simulink model "TwoLVSCSwitch_IGBT"  (R2018a)
settings: Solver=VariableStepAuto  StartTime=0.0  StopTime=0.5  RelTol=1e-3
values from neighbouring files (symbols this model uses):
  C = 1 / (C_pu * omega_base * Z_DC_base)    (= 0.000114731723891)    [ErlingInitialization.m]
  I_base = 2 * S_base / (3 * V_base)    (= 33.3333333333)    [ErlingInitialization.m]
  I_DC_base = S_base / V_DC_base    (= 25)    [ErlingInitialization.m]
  i_load = I_DC_base    (= 25)    [ErlingInitialization.m]
  K_CRCI = K_CRCP / tau    [ErlingInitialization.m]
  K_CRCP = 1 / (C_pu * omega_base * sqrt(tau * tau_eq))    [ErlingInitialization.m]
  K_i = R_pu / tau_eq    (= 16.6666666667)    [ErlingInitialization.m]
  K_p = L_pu / (omega_base * tau_eq)    (= 0.795774715459)    [ErlingInitialization.m]
  L = L_pu * Z_base / omega_base    (= 0.00572957795131)    [ErlingInitialization.m]
  L_pu = 0.15    [ErlingInitialization.m]
  R = R_pu * Z_base    (= 0.12)    [ErlingInitialization.m]
  tau_PWM = 1 / 10000    (= 0.0001)    [ErlingInitialization.m]
  Ts = 1e-6    (= 1e-06)    [ErlingInitialization.m]
  V_base = 400    [ErlingInitialization.m]
  V_DC_base = V_base * 2    (= 800)    [ErlingInitialization.m]
  V_DC_start = V_DC_base    (= 800)    [ErlingInitialization.m]
libraries: powerlib x17
settings Model: Creator=nartgnilre  LastModifiedBy=nartgnilre

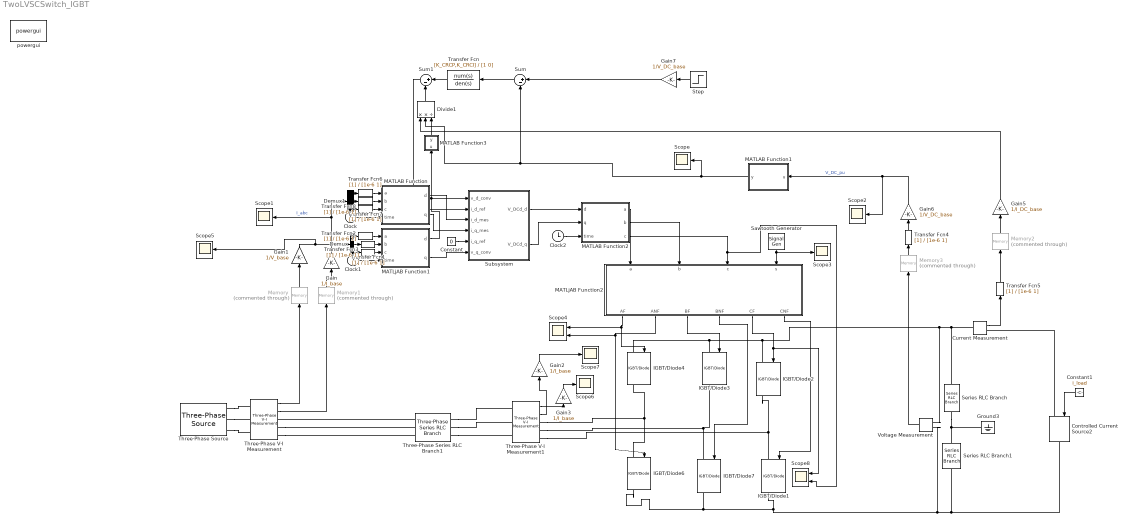
== system TwoLVSCSwitch_IGBT ==
  Clock : Clock
  Clock1 : Clock
  Clock2 : Clock
  Constant : Constant  Value=0
  Constant1 : Constant  Value=i_load
  Controlled Current Source2 : powerlib/Electrical Sources/Controlled Current Source  Initialize=on  Source_Type=AC  Amplitude=0  Phase=0  Frequency=0  Measurements=None
  Current Measurement : powerlib/Measurements/Current Measurement  PhasorSimulation=off  OutputType=Magnitude  PSBequivalent=0
  Demux : Demux  Outputs=3
  Demux1 : Demux  Outputs=3
  Divide1 : Product  Inputs=**/
  Gain : Gain  Gain=1/I_base
  Gain1 : Gain  Gain=1/V_base
  Gain2 : Gain  Gain=1/I_base
  Gain3 : Gain  Gain=1/I_base
  Gain5 : Gain  Gain=1/I_DC_base
  Gain6 : Gain  Gain=1/V_DC_base
  Gain7 : Gain  Gain=1/V_DC_base
  Ground3 : powerlib/Elements/Ground  LConnTagsString=a
  IGBT/Diode{1..4,6..7} (6 alike) : powerlib/Power Electronics/IGBT//Diode  Ron=1e-5  Rs=1e5  Cs=inf  Measurements=on
  MATLAB Function : MATLAB Function  TreatAsAtomicUnit=on
  MATLAB Function1 : MATLAB Function  TreatAsAtomicUnit=on
  MATLAB Function2 : MATLAB Function  TreatAsAtomicUnit=on
  MATLAB Function3 : MATLAB Function  TreatAsAtomicUnit=on
  MATLjAB Function1 : MATLAB Function  TreatAsAtomicUnit=on
  MATLjAB Function2 : MATLAB Function  TreatAsAtomicUnit=on
  Memory : Memory  Commented=through  InitialCondition=V_base
  Memory1 : Memory  Commented=through  InitialCondition=I_base
  Memory2 : Memory  Commented=through  InitialCondition=I_base
  Memory3 : Memory  Commented=through  InitialCondition=V_base
  Sawtooth Generator : SignalGenerator  WaveForm=sawtooth  Frequency=1/tau_PWM
  Scope{,1..3,5..7} (7 alike) : Scope
  Scope4 : Scope  NumInputPorts=2
  Scope8 : Scope  NumInputPorts=2
  Series RLC Branch : powerlib/Elements/Series RLC Branch  LConnTagsString=__new0  RConnTagsString=__new0  BranchType=C  Resistance=1  Inductance=1e-3  SetiL0=off  InitialCurrent=0  Capacitance=2*C  Setx0=on  InitialVoltage=V_DC_start/2  Measurements=None
  Series RLC Branch1 : powerlib/Elements/Series RLC Branch  LConnTagsString=__new0  RConnTagsString=__new0  BranchType=C  Resistance=1  Inductance=1e-3  SetiL0=off  InitialCurrent=0  Capacitance=2*C  Setx0=on  InitialVoltage=-V_DC_start/2  Measurements=None
  Step : Step  Time=0.4  Before=V_DC_start*1.2  After=V_DC_start*1.3  SampleTime=0
  Subsystem : Subsystem
  Sum : Sum  Inputs=|+-
  Sum1 : Sum  Inputs=|+-
  Three-Phase Series RLC Branch1 : powerlib/Elements/Three-Phase Series RLC Branch  LConnTagsString=A|B|C  RConnTagsString=A|B|C  BranchType=RL  Resistance=R  Inductance=L  Capacitance=0  Measurements=Branch voltages and currents
  Three-Phase V-I Measurement : powerlib/Measurements/Three-Phase V-I Measurement  VoltageMeasurement=phase-to-ground  SetLabelV=off  LabelV=Vabc  Vpu=off  VpuLL=off  CurrentMeasurement=yes  SetLabelI=off  LabelI=Iabc  Ipu=off  Pbase=S_base  Vbase=V_base  OutputType=Complex  PhasorSimulation=off  PSBequivalent=0
  Three-Phase V-I Measurement1 : powerlib/Measurements/Three-Phase V-I Measurement  VoltageMeasurement=phase-to-ground  SetLabelV=off  LabelV=Vabc  Vpu=off  VpuLL=off  CurrentMeasurement=yes  SetLabelI=off  LabelI=Iabc  Ipu=off  Pbase=S_base  Vbase=V_base  OutputType=Complex  PhasorSimulation=off  PSBequivalent=0
  Three-Phase Source : powerlib/Electrical Sources/Three-Phase Source  InternalConnection=Yg  VoltagePhases=off  Voltage=V_base*sqrt(3)/sqrt(2)  PhaseAngle=90  Voltage_phases=[25e3 25e3 25e3]/sqrt(3)  PhaseAngles_phases=[0 -120 +120]  Frequency=50  NonIdealSource=off  SpecifyImpedance=off  Resistance=0.8929  Inductance=16.58e-3  ShortCircuitLevel=100e6  BaseVoltage=25e3  XRratio=7  BusType=swing  Pref=10e3  Qref=0  Prefabc=[10e3, 10e3, 10e3]  Qrefabc=[0, 0, 0]  Qmin=-inf  Qmax=inf
      settings: SourceProductName=Simscape Electrical
  Transfer Fcn : TransferFcn  Numerator=[K_CRCP,K_CRCI]  Denominator=[1 0]
  Transfer Fcn{1..8} (8 alike) : TransferFcn  Denominator=[1e-6 1]
  Voltage Measurement : powerlib/Measurements/Voltage Measurement  PhasorSimulation=off  OutputType=Magnitude  PSBequivalent=0
  powergui : powerlib/powergui  Priority=1  SimulationMode=Discrete  SampleTime=Ts  frequency=60  Iterations=50  frequencyindice=0  Pbase=100e6  ErrMax=1e-4  UnitsV=kV  UnitsW=MW  buscounter=0  FunctionMessages=off  echomessages=off  EnableUseOfTLC=off  CurrentSourceSwitches=off  DisableSnubberDevices=off  DisableRonSwitches=off  DisableVfSwitches=off  DisplayEquations=off  SolverType=Tustin/Backward Euler (TBE)  Interpol=off  ExternalGateDelay=off  methode=off  Ts=100  x0status=blocks  SPID=off  SwTol=0  HookPort=off  RestoreLinks=warning  ResistiveCurrentMeasurement=off  Frange=[0:2:500]  Ylog=off  Xlog=on  ShowGrid=off  save=off  variable=ZData  structure=0  ZoomFFT=off  StartTime=0.0  cycles=1  DisplayStyle=1  fundamental=60  FreqAxis=off  MaxFrequency=1000  frequencyindicesteady=1  RmsSteady=1  display=off
  wires:
  Gain3/1 -> Scope6/1
  Gain6/1 -> Scope2/1, MATLAB Function1/1(u)  "V_DC_pu"
  MATLjAB Function1/2(q) -> Subsystem/6(v_q_conv)
  MATLjAB Function2/6(CNF) -> IGBT/Diode1/1
  Clock1/1 -> MATLjAB Function1/4(time)
  Demux1/2 -> Transfer Fcn7/1
  Demux/1 -> Transfer Fcn2/1
  Transfer Fcn6/1 -> MATLAB Function/1(a)
  MATLAB Function2/2(b) -> MATLjAB Function2/2(b)
  Sawtooth Generator/1 -> MATLjAB Function2/4(s), Scope3/1
  MATLjAB Function2/4(BNF) -> IGBT/Diode7/1
  Step/1 -> Gain7/1
  Transfer Fcn4/1 -> Gain6/1
  Gain/1 -> Scope1/1, Demux1/1  "I_abc"
  Demux/3 -> Transfer Fcn3/1
  MATLAB Function2/3(c) -> Scope8/2, MATLjAB Function2/3(c)
  Gain1/1 -> Scope5/1, Demux/1
  Transfer Fcn5/1 -> Memory2/1
  Sum/1 -> Transfer Fcn/1
  Memory2/1 -> Gain5/1
  Divide1/1 -> Sum1/2
  Demux/2 -> Transfer Fcn1/1
  Transfer Fcn3/1 -> MATLjAB Function1/3(c)
  Sum1/1 -> Subsystem/2(i_d_ref)
  Three-Phase V-I Measurement1/1 -> Gain3/1
  Gain2/1 -> Scope7/1
  MATLjAB Function2/3(BF) -> IGBT/Diode3/1
  Three-Phase V-I Measurement1/2 -> Gain2/1
  Transfer Fcn7/1 -> MATLAB Function/2(b)
  Three-Phase V-I Measurement/1 -> Memory/1
  Demux1/1 -> Transfer Fcn6/1
  MATLAB Function2/1(a) -> MATLjAB Function2/1(a)
  MATLAB Function/1(d) -> Subsystem/3(i_d_mes)
  Gain7/1 -> Sum/1
  Transfer Fcn/1 -> Sum1/1
  Subsystem/1(V_DCd_d) -> MATLAB Function2/1(d)
  Transfer Fcn1/1 -> MATLjAB Function1/2(b)
  Three-Phase V-I Measurement/2 -> Memory1/1
  Clock2/1 -> MATLAB Function2/3(time)
  MATLAB Function1/1(y) -> Sum/2, Divide1/2, Scope/1
  Memory3/1 -> Transfer Fcn4/1
  Memory1/1 -> Gain/1
  MATLAB Function/2(q) -> Subsystem/4(i_q_mes)
  Clock/1 -> MATLAB Function/4(time)
  Constant1/1 -> Controlled Current Source2/1
  Subsystem/2("V_DCd_q ") -> MATLAB Function2/2(q)
  Voltage Measurement/1 -> Memory3/1
  Transfer Fcn8/1 -> MATLAB Function/3(c)
  Memory/1 -> Gain1/1
  MATLjAB Function1/1(d) -> Subsystem/1("v_d_conv "), MATLAB Function3/1(u)
  MATLjAB Function2/1(AF) -> IGBT/Diode4/1, Scope4/1
  Transfer Fcn2/1 -> MATLjAB Function1/1(a)
  Constant/1 -> Subsystem/5(i_q_ref)
  Current Measurement/1 -> Transfer Fcn5/1
  MATLjAB Function2/2(ANF) -> IGBT/Diode6/1, Scope4/2
  Gain5/1 -> Divide1/1
  Demux1/3 -> Transfer Fcn8/1
  MATLAB Function3/1(y) -> Divide1/3
  MATLjAB Function2/5(CF) -> Scope8/1, IGBT/Diode2/1
  connections:
  Voltage Measurement/LConn1 -- IGBT/Diode4/LConn1 -- IGBT/Diode3/LConn1 -- IGBT/Diode2/LConn1 -- Series RLC Branch/LConn1 -- Current Measurement/LConn1
  IGBT/Diode6/LConn1 -- IGBT/Diode4/RConn1 -- Three-Phase V-I Measurement1/RConn1
  Series RLC Branch/RConn1 -- Ground3/LConn1 -- Series RLC Branch1/RConn1
  IGBT/Diode2/RConn1 -- IGBT/Diode1/LConn1 -- Three-Phase V-I Measurement1/RConn3
  Three-Phase V-I Measurement1/RConn2 -- IGBT/Diode7/LConn1 -- IGBT/Diode3/RConn1
  IGBT/Diode6/RConn1 -- IGBT/Diode7/RConn1 -- IGBT/Diode1/RConn1 -- Series RLC Branch1/LConn1 -- Controlled Current Source2/RConn1 -- Voltage Measurement/LConn2
  Three-Phase Source/RConn1 -- Three-Phase V-I Measurement/LConn1
  Three-Phase V-I Measurement/RConn3 -- Three-Phase Series RLC Branch1/LConn3
  Three-Phase Series RLC Branch1/RConn3 -- Three-Phase V-I Measurement1/LConn3
  Three-Phase Series RLC Branch1/RConn1 -- Three-Phase V-I Measurement1/LConn1
  Controlled Current Source2/LConn1 -- Current Measurement/RConn1
  Three-Phase Series RLC Branch1/RConn2 -- Three-Phase V-I Measurement1/LConn2
  Three-Phase Source/RConn3 -- Three-Phase V-I Measurement/LConn3
  Three-Phase V-I Measurement/RConn2 -- Three-Phase Series RLC Branch1/LConn2
  Three-Phase Source/RConn2 -- Three-Phase V-I Measurement/LConn2
  Three-Phase Series RLC Branch1/LConn1 -- Three-Phase V-I Measurement/RConn1

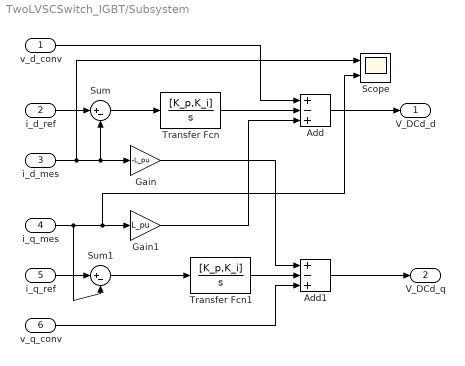
== system TwoLVSCSwitch_IGBT/Subsystem ==
  "v_d_conv " : Inport
  i_d_ref : Inport  Port=2
  i_d_mes : Inport  Port=3
  i_q_mes : Inport  Port=4
  i_q_ref : Inport  Port=5
  v_q_conv : Inport  Port=6
  Add : Sum  Inputs=+-+
  Add1 : Sum  Inputs=+-+
  Gain : Gain  Gain=-L_pu
  Gain1 : Gain  Gain=L_pu
  Scope : Scope  NumInputPorts=2
  Sum : Sum  Inputs=|+-
  Sum1 : Sum  Inputs=|+-
  Transfer Fcn : TransferFcn  Numerator=[K_p,K_i]  Denominator=[1 0]
  Transfer Fcn1 : TransferFcn  Numerator=[K_p,K_i]  Denominator=[1 0]
  V_DCd_d : Outport
  "V_DCd_q " : Outport  Port=2
  wires:
  i_d_ref/1 -> Sum/1
  i_q_ref/1 -> Sum1/1
  i_q_mes/1 -> Scope/2, Gain1/1, Sum1/2
  i_d_mes/1 -> Scope/1, Gain/1, Sum/2
  Sum/1 -> Transfer Fcn/1
  Sum1/1 -> Transfer Fcn1/1
  Transfer Fcn/1 -> Add/2
  Transfer Fcn1/1 -> Add1/2
  Gain/1 -> Add1/1
  v_q_conv/1 -> Add1/3
  Gain1/1 -> Add/3
  "v_d_conv "/1 -> Add/1
  Add1/1 -> "V_DCd_q "/1
  Add/1 -> V_DCd_d/1

== matlab function TwoLVSCSwitch_IGBT/MATLjAB Function1 ==
  data: a input; d output; b input; c input; q output; time input
function [d,q] = abc2dqz(a,b,c,time)
w = 2*pi*50;
d = 2 / 3 * (a * cos(w * time) + b * cos(w * time - 2 * pi / 3) + c * cos(w * time + 2 * pi / 3));
q = 2 / 3 * ((-a * sin(w * time)) - b * sin(w * time - 2 * pi / 3) - c * sin(w * time + 2 * pi / 3));
end

== matlab function TwoLVSCSwitch_IGBT/MATLAB Function ==
  data: a input; d output; b input; c input; q output; time input
function [d,q] = abc2dqz(a,b,c,time)
w = 2*pi*50;
d = 2 / 3 * (a * cos(w * time) + b * cos(w * time - 2 * pi / 3) + c * cos(w * time + 2 * pi / 3));
q = 2 / 3 * ((-a * sin(w * time)) - b * sin(w * time - 2 * pi / 3) - c * sin(w * time + 2 * pi / 3));
end

== matlab function TwoLVSCSwitch_IGBT/MATLAB Function2 ==
  data: d input; a output; q input; b output; time input; c output
function [a,b,c] = dqz2abc(d,q,time)
w = 2*pi*50;
a = d * cos(w * time) - q * sin(w * time);
b = d * cos(w * time - 2 * pi / 3) - q * sin(w * time - 2 * pi / 3);
c = d * cos(w * time + 2 * pi / 3) - q * sin(w * time + 2 * pi / 3);
end

== matlab function TwoLVSCSwitch_IGBT/MATLAB Function1 ==
  data: u input; y output
function y = fcn(u)
if u == 0
    y = 0.01;
else
    y = u;
end
end

== matlab function TwoLVSCSwitch_IGBT/MATLAB Function3 ==
  data: u input; y output
function y = fcn(u)
if u == 0
    y = 0.01;
else
    y = u;
end
end

== matlab function TwoLVSCSwitch_IGBT/MATLjAB Function2 ==
  data: a input; AF output; ANF output; BF output; BNF output; b input; c input; s input; CF output; CNF output
function [AF,ANF,BF,BNF,CF,CNF] = PWM(a,b,c,s)
af = a>s;
bf = b>s;
cf = c>s;
anf = ~af;
bnf = ~bf;
cnf = ~cf;
AF = int16(af);
ANF = int16(anf);
BF = int16(bf);
BNF = int16(bnf);
CF = int16(cf);
CNF = int16(cnf);
end
